simulink model "CornerDetection"  (R2022a)
settings: Solver=FixedStepDiscrete  StartTime=0.0  StopTime=Ts_240p*5  RelTol=1e-3
InitFcn:
  | Ts = 1e-3;
  | Ts_240p = 402*324*Ts;
  | Ts_480p = 525*800*Ts;
undefined symbols (not defined in the file): fspecial, gray, Rec, SDTV
libraries: hdlsllib x8, visionhdlfilter x5, visionhdlio x2, simulink x1, visionhdlutilities x1, visionhdlconversions x1, dspvision x1
settings Model: DataTypeOverride=Off  ModifiedByFormat=The MathWorks Inc.  Creator=The MathWorks, Inc.  LastModifiedBy=The MathWorks Inc.
settings SolverCC: AlgebraicLoopSolver=TrustRegion
settings DataIOCC: LimitDataPoints=on  SaveFormat=Array  SaveOutput=off  SaveTime=off  ReturnWorkspaceOutputs=off
settings OptimizationCC: BlockReduction=off  ConditionallyExecuteInputs=off  DefaultParameterBehavior=Inlined  LifeSpan=inf
settings DebuggingCC: AlgebraicLoopMsg=error  SolverPrmCheckMsg=warning  SingleTaskRateTransMsg=error  ParameterPrecisionLossMsg=none  UnconnectedInputMsg=warning  UnconnectedOutputMsg=warning  UnconnectedLineMsg=warning  AllowSymbolicDim=off  SFUnexpectedBacktrackingDiag=warning  SFNoUnconditionalDefaultTransitionDiag=warning  SFExecutionAtInitializationDiag=none  SFMachineParentedDataDiag=warning  IntegerSaturationMsg=none  ArithmeticOperatorsInVariantConditions=warning
settings HardwareCC: ProdBitPerPointer=32  ProdBitPerSizeT=32  ProdBitPerPtrDiffT=32  ProdLargestAtomicFloat=None  ProdIntDivRoundTo=Undefined  ProdEndianess=Unspecified  ProdWordSize=32  ProdHWDeviceType=ASIC/FPGA->ASIC/FPGA  ProdEqTarget=off
settings ModelReferenceCC: PropagateSignalLabelsOutOfModel=off
settings SFSimCC: SimUseLocalCustomCode=off  CustomCodeUndefinedFunction=UseInterfaceOnly
settings RTWCC: RTWUseLocalCustomCode=off
settings CodeAppCC: StateflowObjectComments=on
settings GRTTargetCC: TargetLangStandard=C89/C90 (ANSI)
settings ConfigComp: CovMetricSettings=dw  CovSaveCumulativeToWorkspaceVar=on  CovSaveSingleToWorkspaceVar=on  CovExternalEMLEnable=off  CovSFcnEnable=off

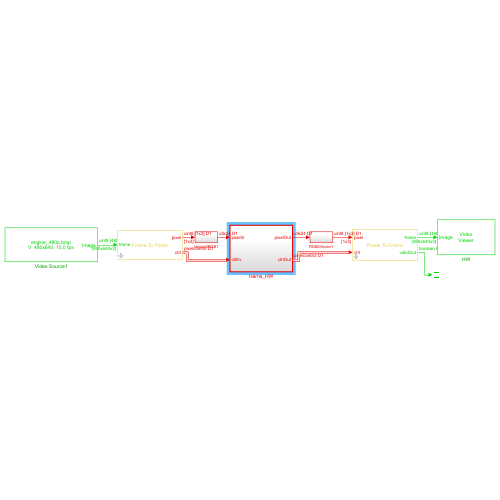
[thumbnail: Simulink's stored preview of the top-level diagram]
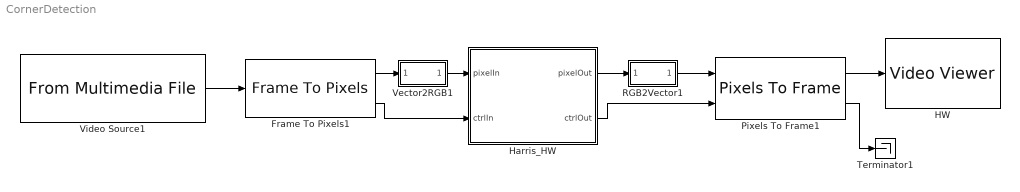
== system CornerDetection ==
  Frame To Pixels1 : visionhdlio/Frame To Pixels  NumComponents=3  NumPixels=1  VideoFormat=480p  ActivePixelsPerLine=640  ActiveVideoLines=480  TotalPixelsPerLine=800  TotalVideoLines=525  StartingActiveLine=36  FrontPorch=16  SampleTime=0  VideoFormatCache=480p  ActivePixelsPerLineCache=32  ActiveVideoLinesCache=18  TotalPixelsPerLineCache=42  TotalVideoLinesCache=28  StartingActiveLineCache=6  FrontPorchCache=5
      settings: SourceProductBaseCode=VT
  HW : VideoViewer  colormapValue=gray(256)  FigPos=[834 788 688 515]
  Harris_HW : Subsystem  TreatAsAtomicUnit=on
  Pixels To Frame1 : visionhdlio/Pixels To Frame  NumComponents=3  NumPixels=1  VideoFormat=480p  ActivePixelsPerLine=640  ActiveVideoLines=480  TotalPixelsPerLine=800  TotalVideoLines=525  VideoFormatCache=480p  ActivePixelsPerLineCache=32  ActiveVideoLinesCache=18  TotalPixelsPerLineCache=42  TotalVideoLinesCache=28
      settings: SourceProductBaseCode=VT
  RGB2Vector1 : Subsystem
  Terminator1 : Terminator
  Vector2RGB1 : Subsystem
  Video Source1 : dspvision/From Multimedia File  inputFilename=D:\datasets\test_images\engine_480p.bmp  readRange=[1 Inf]  loop=on  numPlays=inf  outputStreams=Video only  videoDataType=uint8  audioDataType=int16  inheritSampleTime=off  userDefinedSampleTime=1/15  noAudioOutput=off  isIntensityVideo=off  fourcc=RGB  colorVideoFormat=One multidimensional signal  outputEOF=off  dataOrg=Column-major  audioFrameSize=1024  computeAudioFrameSize=off  outSamplingMode=Sample based
  wires:
  Harris_HW/1(pixelOut) -> RGB2Vector1/1(RGB)
  RGB2Vector1/1(RGBVector) -> Pixels To Frame1/1
  Pixels To Frame1/2 -> Terminator1/1
  Frame To Pixels1/2 -> Harris_HW/2(ctrlIn)
  Harris_HW/2(ctrlOut) -> Pixels To Frame1/2
  Frame To Pixels1/1 -> Vector2RGB1/1(RGBVector)
  Vector2RGB1/1(RGB) -> Harris_HW/1(pixelIn)
  Video Source1/1 -> Frame To Pixels1/1
  Pixels To Frame1/1 -> HW/1

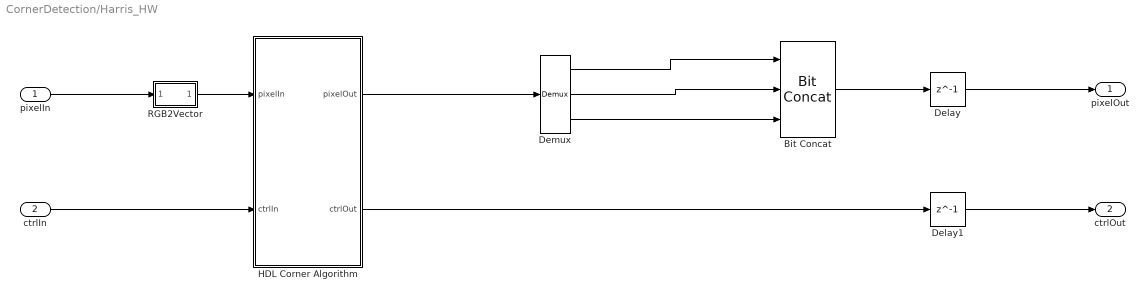
== system CornerDetection/Harris_HW ==
  pixelIn : Inport
  ctrlIn : Inport  Port=2
  Bit Concat : hdlsllib/Logic and Bit Operations/Bit Concat  numInputs=3
  Delay : Delay  DelayLength=1  InitialCondition=0
  Delay1 : Delay  DelayLength=1  InitialCondition=0
  Demux : Demux  Outputs=3
  HDL Corner Algorithm : Subsystem  TreatAsAtomicUnit=on
  RGB2Vector : Subsystem
  pixelOut : Outport  VectorParamsAs1DForOutWhenUnconnected=off
  ctrlOut : Outport  Port=2  VectorParamsAs1DForOutWhenUnconnected=off
  wires:
  ctrlIn/1 -> HDL Corner Algorithm/2(ctrlIn)
  pixelIn/1 -> RGB2Vector/1(RGB)
  RGB2Vector/1(RGBVector) -> HDL Corner Algorithm/1(pixelIn)
  Bit Concat/1 -> Delay/1
  HDL Corner Algorithm/2(ctrlOut) -> Delay1/1
  HDL Corner Algorithm/1(pixelOut) -> Demux/1
  Demux/1 -> Bit Concat/1
  Demux/2 -> Bit Concat/2
  Demux/3 -> Bit Concat/3
  Delay/1 -> pixelOut/1
  Delay1/1 -> ctrlOut/1

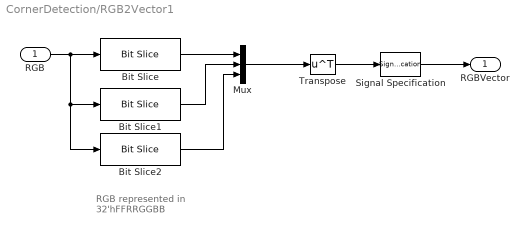
== system CornerDetection/RGB2Vector1 ==
  note: RGB represented in
      | 32'hFFRRGGBB
  RGB : Inport
  Bit Slice : hdlsllib/Logic and Bit Operations/Bit Slice  lidx=23  ridx=16
      settings: SourceProductBaseCode=SL
  Bit Slice1 : hdlsllib/Logic and Bit Operations/Bit Slice  lidx=15  ridx=8
      settings: SourceProductBaseCode=SL
  Bit Slice2 : hdlsllib/Logic and Bit Operations/Bit Slice  lidx=7  ridx=0
      settings: SourceProductBaseCode=SL
  Mux : Mux  Inputs=3
  Signal Specification : SignalSpecification
  Transpose : Math  Operator=transpose  SignedPower=on
  RGBVector : Outport  VectorParamsAs1DForOutWhenUnconnected=off
  wires:
  Mux/1 -> Transpose/1
  Bit Slice/1 -> Mux/1
  Bit Slice2/1 -> Mux/3
  Bit Slice1/1 -> Mux/2
  RGB/1 -> Bit Slice2/1, Bit Slice1/1, Bit Slice/1
  Transpose/1 -> Signal Specification/1
  Signal Specification/1 -> RGBVector/1

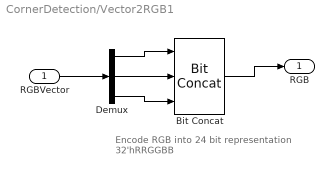
== system CornerDetection/Vector2RGB1 ==
  note: Encode RGB into 24 bit representation
      | 32'hRRGGBB
  RGBVector : Inport
  Bit Concat : hdlsllib/Logic and Bit Operations/Bit Concat  numInputs=3
  Demux : Demux  Outputs=3
  RGB : Outport  VectorParamsAs1DForOutWhenUnconnected=off
  wires:
  Bit Concat/1 -> RGB/1
  RGBVector/1 -> Demux/1
  Demux/1 -> Bit Concat/1
  Demux/2 -> Bit Concat/2
  Demux/3 -> Bit Concat/3

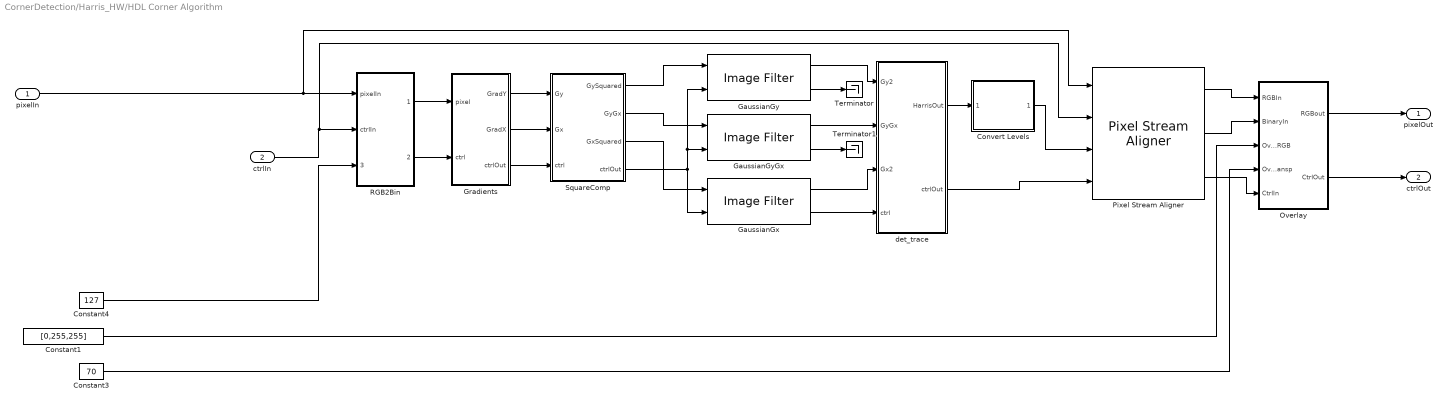
== system CornerDetection/Harris_HW/HDL Corner Algorithm ==
  pixelIn : Inport
  ctrlIn : Inport  Port=2
  Constant1 : Constant  Value=[0,255,255]  VectorParams1D=off  OutDataTypeStr=uint8  SampleTime=-1
  Constant3 : Constant  Value=70  OutDataTypeStr=uint8  SampleTime=-1
  Constant4 : Constant  Value=127  OutDataTypeStr=uint8  SampleTime=-1
  Convert Levels : Subsystem
  GaussianGx : visionhdlfilter/Image Filter  CoefficientsSource=Property  Coefficients=fspecial('gaussian',[5,5],1.5)  PaddingMethod=Constant  PaddingValue=0  LineBufferSize=1024  SimulateUsing=Code generation  roundingMode=Floor  overflowMode=off  CoeffDataTypeStr=fixdt(1,18,21)  CoeffMin=[]  CoeffMax=[]  OutputMin=[]  OutputMax=[]
      settings: SourceProductBaseCode=VT
  GaussianGy : visionhdlfilter/Image Filter  CoefficientsSource=Property  Coefficients=fspecial('gaussian',[5,5],1.5)  PaddingMethod=Constant  PaddingValue=0  LineBufferSize=1024  SimulateUsing=Code generation  roundingMode=Floor  overflowMode=off  CoeffDataTypeStr=fixdt(1,18,21)  CoeffMin=[]  CoeffMax=[]  OutputMin=[]  OutputMax=[]
      settings: SourceProductBaseCode=VT
  GaussianGyGx : visionhdlfilter/Image Filter  CoefficientsSource=Property  Coefficients=fspecial('gaussian',[5,5],1.5)  PaddingMethod=Constant  PaddingValue=0  LineBufferSize=1024  SimulateUsing=Code generation  roundingMode=Floor  overflowMode=off  CoeffDataTypeStr=fixdt(1,18,21)  CoeffMin=[]  CoeffMax=[]  OutputMin=[]  OutputMax=[]
      settings: SourceProductBaseCode=VT
  Gradients : Subsystem
  Overlay : Subsystem
  Pixel Stream Aligner : visionhdlutilities/Pixel Stream Aligner  LineBufferSize=1024  MaximumNumberOfLines=10  SimulateUsing=Code generation
      settings: SourceProductBaseCode=VT
  RGB2Bin : Subsystem
  SquareComp : Subsystem
  Terminator : Terminator
  Terminator1 : Terminator
  det_trace : Subsystem
  pixelOut : Outport  VectorParamsAs1DForOutWhenUnconnected=off
  ctrlOut : Outport  Port=2  VectorParamsAs1DForOutWhenUnconnected=off
  wires:
  Constant4/1 -> RGB2Bin/3(SliceLevel)
  RGB2Bin/2(ctrlOut) -> Gradients/2(ctrl)
  RGB2Bin/1(pixelOut) -> Gradients/1(pixel)
  det_trace/1(HarrisOut) -> Convert Levels/1(HarrisIn)
  Constant3/1 -> Overlay/4(OverlayTransp)
  Gradients/3(ctrlOut) -> SquareComp/3(ctrl)
  Gradients/2(GradX) -> SquareComp/2(Gx)
  Gradients/1(GradY) -> SquareComp/1(Gy)
  ctrlIn/1 -> Pixel Stream Aligner/2, RGB2Bin/2(ctrlIn)
  GaussianGx/2 -> det_trace/4(ctrl)
  GaussianGx/1 -> det_trace/3(Gx2)
  GaussianGyGx/1 -> det_trace/2(GyGx)
  GaussianGy/1 -> det_trace/1(Gy2)
  SquareComp/3(GxSquared) -> GaussianGx/1
  SquareComp/2(GyGx) -> GaussianGyGx/1
  SquareComp/1(GySquared) -> GaussianGy/1
  SquareComp/4(ctrlOut) -> GaussianGx/2, GaussianGy/2, GaussianGyGx/2
  GaussianGyGx/2 -> Terminator1/1
  GaussianGy/2 -> Terminator/1
  Pixel Stream Aligner/1 -> Overlay/1(RGBIn)
  Pixel Stream Aligner/2 -> Overlay/2(BinaryIn)
  Pixel Stream Aligner/3 -> Overlay/5(CtrlIn)
  Constant1/1 -> Overlay/3(OverlayRGB)
  pixelIn/1 -> Pixel Stream Aligner/1, RGB2Bin/1(pixelIn)
  Convert Levels/1(PixelOut) -> Pixel Stream Aligner/3
  det_trace/2(ctrlOut) -> Pixel Stream Aligner/4
  Overlay/1(RGBout) -> pixelOut/1
  Overlay/2("CtrlOut ") -> ctrlOut/1

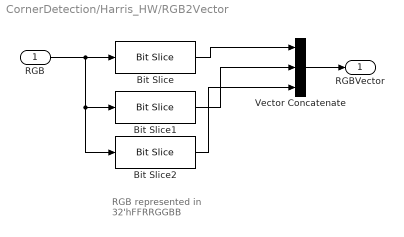
== system CornerDetection/Harris_HW/RGB2Vector ==
  note: RGB represented in
      | 32'hFFRRGGBB
  RGB : Inport
  Bit Slice : hdlsllib/Logic and Bit Operations/Bit Slice  lidx=23  ridx=16
      settings: SourceProductBaseCode=SL
  Bit Slice1 : hdlsllib/Logic and Bit Operations/Bit Slice  lidx=15  ridx=8
      settings: SourceProductBaseCode=SL
  Bit Slice2 : hdlsllib/Logic and Bit Operations/Bit Slice  lidx=7  ridx=0
      settings: SourceProductBaseCode=SL
  Vector Concatenate : Concatenate  NumInputs=3  Mode=Multidimensional array  ConcatenateDimension=2
  RGBVector : Outport  VectorParamsAs1DForOutWhenUnconnected=off
  wires:
  Bit Slice/1 -> Vector Concatenate/1
  Bit Slice2/1 -> Vector Concatenate/3
  Bit Slice1/1 -> Vector Concatenate/2
  RGB/1 -> Bit Slice2/1, Bit Slice1/1, Bit Slice/1
  Vector Concatenate/1 -> RGBVector/1

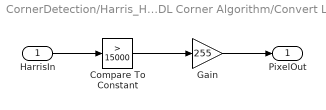
== system CornerDetection/Harris_HW/HDL Corner Algorithm/Convert Levels ==
  HarrisIn : Inport
  Compare To Constant : simulink/Logic and Bit Operations/Compare To Constant  relop=>  const=15000  OutDataTypeStr=uint8
  Gain : Gain  Gain=255  OutDataTypeStr=uint8
  PixelOut : Outport  VectorParamsAs1DForOutWhenUnconnected=off
  wires:
  Gain/1 -> PixelOut/1
  HarrisIn/1 -> Compare To Constant/1
  Compare To Constant/1 -> Gain/1

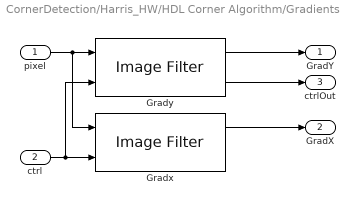
== system CornerDetection/Harris_HW/HDL Corner Algorithm/Gradients ==
  pixel : Inport
  ctrl : Inport  Port=2
  Gradx : visionhdlfilter/Image Filter  CoefficientsSource=Property  Coefficients=[0,0,0;1, 0,-1;0,0,0]  PaddingMethod=Replicate  PaddingValue=0  LineBufferSize=1024  SimulateUsing=Code generation  roundingMode=Floor  overflowMode=off  CoeffDataTypeStr=fixdt(1,2,0)  CoeffMin=[]  CoeffMax=[]  OutputDataTypeStr=fixdt(1,9,0)  OutputMin=[]  OutputMax=[]
      settings: SourceProductBaseCode=VT
  Grady : visionhdlfilter/Image Filter  CoefficientsSource=Property  Coefficients=[0,1,0; 0,0,0; 0,-1,0]  PaddingMethod=Replicate  PaddingValue=0  LineBufferSize=1024  SimulateUsing=Code generation  roundingMode=Floor  overflowMode=off  CoeffDataTypeStr=fixdt(1,2,0)  CoeffMin=[]  CoeffMax=[]  OutputDataTypeStr=fixdt(1,9,0)  OutputMin=[]  OutputMax=[]
      settings: SourceProductBaseCode=VT
  GradY : Outport  VectorParamsAs1DForOutWhenUnconnected=off
  GradX : Outport  Port=2  VectorParamsAs1DForOutWhenUnconnected=off
  ctrlOut : Outport  Port=3  VectorParamsAs1DForOutWhenUnconnected=off
  wires:
  Grady/2 -> ctrlOut/1
  Gradx/1 -> GradX/1
  ctrl/1 -> Gradx/2, Grady/2
  pixel/1 -> Grady/1, Gradx/1
  Grady/1 -> GradY/1

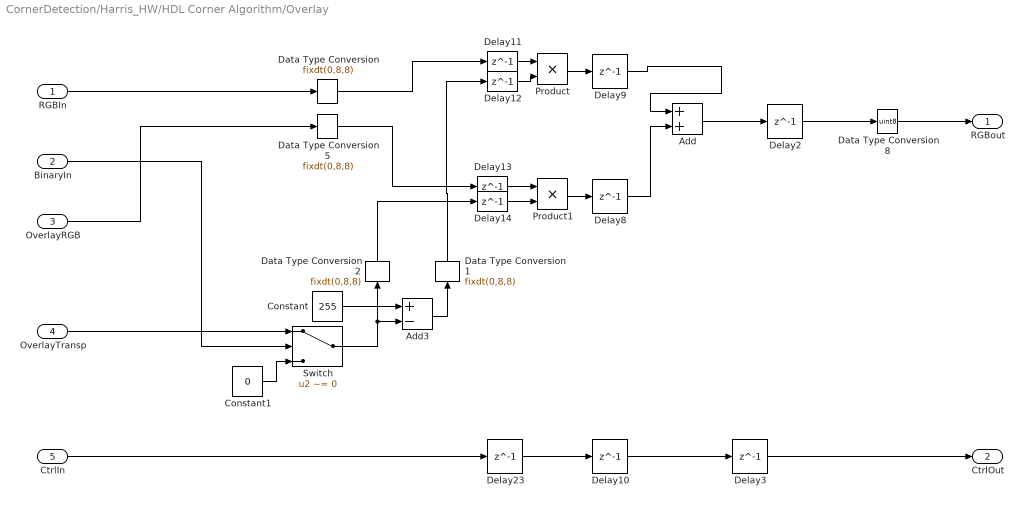
== system CornerDetection/Harris_HW/HDL Corner Algorithm/Overlay ==
  RGBIn : Inport
  BinaryIn : Inport  Port=2
  OverlayRGB : Inport  Port=3
  OverlayTransp : Inport  Port=4
  CtrlIn : Inport  Port=5
  Add : Sum  OutDataTypeStr=fixdt(0,8,8)
  Add3 : Sum  Inputs=+-  OutDataTypeStr=uint8
  Constant : Constant  Value=255  OutDataTypeStr=uint8  SampleTime=-1
  Constant1 : Constant  Value=0  OutDataTypeStr=uint8  SampleTime=-1
  Data Type Conversion{,1..2,5} (4 alike) : DataTypeConversion  OutDataTypeStr=fixdt(0,8,8)  ConvertRealWorld=Stored Integer (SI)  SaturateOnIntegerOverflow=off  RndMeth=Floor
  Data Type Conversion8 : DataTypeConversion  OutDataTypeStr=uint8  ConvertRealWorld=Stored Integer (SI)  SaturateOnIntegerOverflow=off  RndMeth=Floor
  Delay{2..3,8..14,23} (10 alike) : Delay  DelayLength=1
  Product : Product  OutDataTypeStr=fixdt(0,8,8)  SaturateOnIntegerOverflow=on
  Product1 : Product  OutDataTypeStr=fixdt(0,8,8)  SaturateOnIntegerOverflow=on
  Switch : Switch  Criteria=u2 ~= 0  SaturateOnIntegerOverflow=off  InputSameDT=off
  RGBout : Outport  VectorParamsAs1DForOutWhenUnconnected=off
  "CtrlOut " : Outport  Port=2  VectorParamsAs1DForOutWhenUnconnected=off
  wires:
  Add/1 -> Delay2/1
  Constant/1 -> Add3/1
  Add3/1 -> Data Type Conversion1/1
  Switch/1 -> Data Type Conversion2/1, Add3/2
  OverlayTransp/1 -> Switch/1
  BinaryIn/1 -> Switch/2
  Constant1/1 -> Switch/3
  Delay2/1 -> Data Type Conversion8/1
  Delay3/1 -> "CtrlOut "/1
  Product1/1 -> Delay8/1
  Product/1 -> Delay9/1
  Delay8/1 -> Add/2
  Delay10/1 -> Delay3/1
  Delay11/1 -> Product/1
  Delay12/1 -> Product/2
  Delay13/1 -> Product1/1
  Delay14/1 -> Product1/2
  Delay23/1 -> Delay10/1
  CtrlIn/1 -> Delay23/1
  Data Type Conversion/1 -> Delay11/1
  Data Type Conversion1/1 -> Delay12/1
  Data Type Conversion2/1 -> Delay14/1
  OverlayRGB/1 -> Data Type Conversion5/1
  RGBIn/1 -> Data Type Conversion/1
  Data Type Conversion8/1 -> RGBout/1
  Data Type Conversion5/1 -> Delay13/1
  Delay9/1 -> Add/1

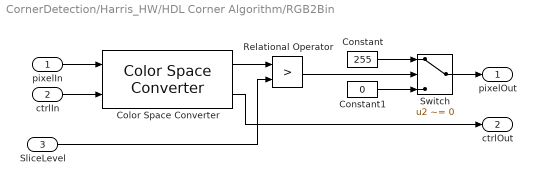
== system CornerDetection/Harris_HW/HDL Corner Algorithm/RGB2Bin ==
  pixelIn : Inport
  ctrlIn : Inport  Port=2
  SliceLevel : Inport  Port=3
  Color Space Converter : visionhdlconversions/Color Space Converter  Conversion=RGB to intensity  ConversionStandard=Rec. 601 (SDTV)  ScanningStandard=1250/50/2:1  SimulateUsing=Code generation
      settings: SourceProductBaseCode=VT
  Constant : Constant  Value=255  OutDataTypeStr=uint8  SampleTime=-1
  Constant1 : Constant  Value=0  OutDataTypeStr=uint8  SampleTime=-1
  Relational Operator : RelationalOperator  Operator=>  OutDataTypeStr=boolean  InputSameDT=off
  Switch : Switch  Criteria=u2 ~= 0  SaturateOnIntegerOverflow=off  InputSameDT=off
  pixelOut : Outport  VectorParamsAs1DForOutWhenUnconnected=off
  ctrlOut : Outport  Port=2  VectorParamsAs1DForOutWhenUnconnected=off
  wires:
  Color Space Converter/2 -> ctrlOut/1
  ctrlIn/1 -> Color Space Converter/2
  pixelIn/1 -> Color Space Converter/1
  Color Space Converter/1 -> Relational Operator/1
  Constant1/1 -> Switch/3
  Constant/1 -> Switch/1
  SliceLevel/1 -> Relational Operator/2
  Relational Operator/1 -> Switch/2
  Switch/1 -> pixelOut/1

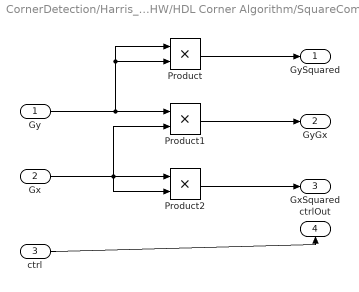
== system CornerDetection/Harris_HW/HDL Corner Algorithm/SquareComp ==
  Gy : Inport
  Gx : Inport  Port=2
  ctrl : Inport  Port=3
  Product : Product
  Product1 : Product
  Product2 : Product
  GySquared : Outport  VectorParamsAs1DForOutWhenUnconnected=off
  GyGx : Outport  Port=2  VectorParamsAs1DForOutWhenUnconnected=off
  GxSquared : Outport  Port=3  VectorParamsAs1DForOutWhenUnconnected=off
  ctrlOut : Outport  Port=4  VectorParamsAs1DForOutWhenUnconnected=off
  wires:
  Gx/1 -> Product2/2, Product2/1, Product1/2
  Gy/1 -> Product1/1, Product/1, Product/2
  Product1/1 -> GyGx/1
  Product/1 -> GySquared/1
  Product2/1 -> GxSquared/1
  ctrl/1 -> ctrlOut/1

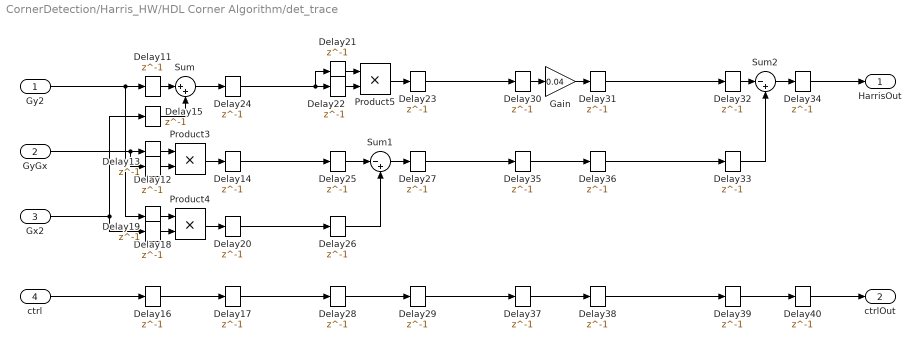
== system CornerDetection/Harris_HW/HDL Corner Algorithm/det_trace ==
  Gy2 : Inport
  GyGx : Inport  Port=2
  Gx2 : Inport  Port=3
  ctrl : Inport  Port=4
  Delay{11..40} (30 alike) : Delay  DelayLength=1  InitialCondition=0
  Gain : Gain  Gain=0.04  ParamDataTypeStr=fixdt(0,16,16)  OutDataTypeStr=Inherit: Same as input
  Product3 : Product
  Product4 : Product
  Product5 : Product
  Sum : Sum  Inputs=|++  OutDataTypeStr=Inherit: Same as first input
  Sum1 : Sum  Inputs=|-+
  Sum2 : Sum  Inputs=|-+
  HarrisOut : Outport  VectorParamsAs1DForOutWhenUnconnected=off
  ctrlOut : Outport  Port=2  VectorParamsAs1DForOutWhenUnconnected=off
  wires:
  Delay33/1 -> Sum2/2
  Gain/1 -> Delay31/1
  Delay16/1 -> Delay17/1
  Delay29/1 -> Delay37/1
  Delay23/1 -> Delay30/1
  Delay40/1 -> ctrlOut/1
  Gy2/1 -> Delay11/1, Delay18/1
  Delay36/1 -> Delay33/1
  Delay37/1 -> Delay38/1
  Sum2/1 -> Delay34/1
  Product4/1 -> Delay20/1
  Delay18/1 -> Product4/1
  Delay32/1 -> Sum2/1
  Delay24/1 -> Delay22/1, Delay21/1
  Delay19/1 -> Product4/2
  Delay14/1 -> Delay25/1
  Sum/1 -> Delay24/1
  Delay35/1 -> Delay36/1
  Delay17/1 -> Delay28/1
  Delay28/1 -> Delay29/1
  GyGx/1 -> Delay12/1, Delay13/1
  Delay27/1 -> Delay35/1
  Delay22/1 -> Product5/2
  Delay34/1 -> HarrisOut/1
  Delay20/1 -> Delay26/1
  Delay39/1 -> Delay40/1
  Delay30/1 -> Gain/1
  Delay21/1 -> Product5/1
  Delay38/1 -> Delay39/1
  Delay25/1 -> Sum1/1
  Sum1/1 -> Delay27/1
  Delay26/1 -> Sum1/2
  Delay11/1 -> Sum/1
  Delay13/1 -> Product3/2
  Product5/1 -> Delay23/1
  ctrl/1 -> Delay16/1
  Delay15/1 -> Sum/2
  Delay12/1 -> Product3/1
  Gx2/1 -> Delay15/1, Delay19/1
  Delay31/1 -> Delay32/1
  Product3/1 -> Delay14/1
